simulink model "testAlphaWallOut"  (R2013b)
settings: Solver=VariableStepDiscrete  StartTime=0.0  StopTime=20  RelTol=1e-3
libraries: carnot x3, simulink x1
settings Model: Creator=drhf  LastModifiedBy=drhf
settings DataIOCC: ReturnWorkspaceOutputs=on
settings OptimizationCC: InlineParams=on
settings DebuggingCC: ReadBeforeWriteMsg=DisableAll  WriteAfterWriteMsg=DisableAll  WriteAfterReadMsg=DisableAll  MultiTaskDSMMsg=none
settings ModelReferenceCC: UpdateModelReferenceTargets=IfOutOfDate
settings SFSimCC: SFSimEcho=off

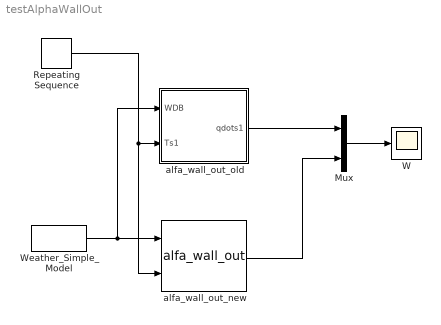
== system testAlphaWallOut ==
  Mux : Mux  Inputs=2
  Repeating Sequence : simulink/Sources/Repeating Sequence  rep_seq_t=[0 10]  rep_seq_y=[10 30]
  W : Scope
  Weather_Simple_Model : carnot/Weather/Weather_Simple_Model  lat=60  Ibn=900  Idg=100  tamb=5  deltaTsky=-6  rh=50  precip="10e-3/24/3600           % 10 mm in 24 h"  cloud=0.125  p=1013e2  vw=1  wdir=270
  alfa_wall_out_new : carnot/Load/Houses/heat_transfer/alfa_wall_out  pos=0  absorption_out=0.4  emission_out=0.7  wallsurface=1
  alfa_wall_out_old : Subsystem  AncestorBlock=carnot/Load/Houses/heat_transfer/alfa_wall_out  mask(ALFA){pos=0, absorption_out=0.4, emission_out=0.7, wallsurface=1}
      mask prompts: pos "Azimut (south = 0, east = -90) in degrees"; absorption_out "Solar absorption outside (0..1)"; emission_out "Longwave emissivity of surface (0..1)"; wallsurface "Wall surface in m²"
      mask help:
      | Convective and radiative HEAT TRANSFER at the WEATHER EXPOSED SURFACE of an OUTER WALL.
      |
      | [W*] : modified weather data, adapted to height over ground,
      | Ts : temperature of outdoor wall surface, °C,
      | qdots : specific heat flow into wall / window construction, W/m^2.
      mask init:
      | if length(pos) == 1
      |     pos = [90  pos 0]; % pos is [inclination azimut rotation]
      | end
  wires:
  Repeating Sequence/1 -> alfa_wall_out_old/2(Ts1), alfa_wall_out_new/2
  alfa_wall_out_old/1(qdots1) -> Mux/1
  alfa_wall_out_new/1 -> Mux/2
  Mux/1 -> W/1
  Weather_Simple_Model/1 -> alfa_wall_out_old/1(WDB), alfa_wall_out_new/1

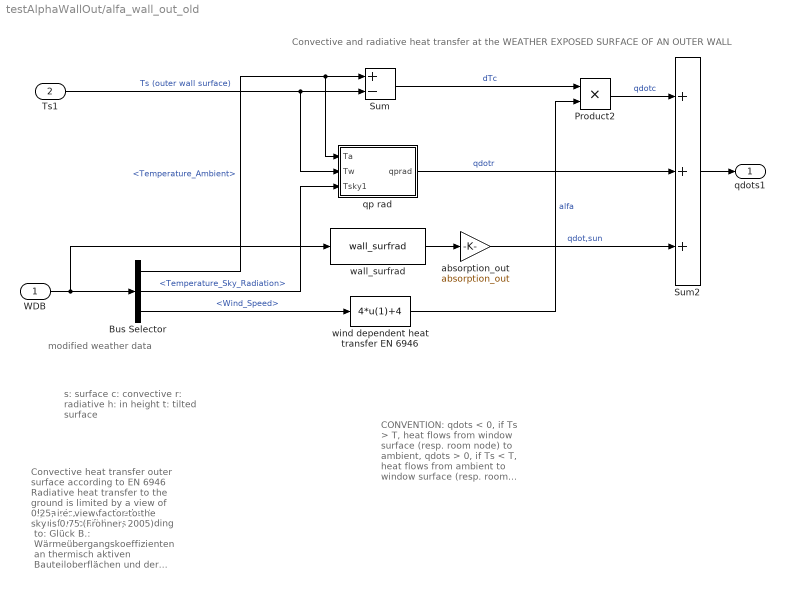
== system testAlphaWallOut/alfa_wall_out_old ==
  note: dynamic, convective heat transfer coefficients according to: Glück B.: Wärmeübergangskoeffizienten an thermisch aktiven Bauteiloberflächen
      | und der Übergang zu Basiskennlinien für die Wärmestromdichte; gi Gesundheits-Ingenieur; 128. Jahrgang 2007, Heft 1, Seiten 1-10
  note: Convective heat transfer outer surface according to EN 6946
      | Radiative heat transfer to the ground is limited by a view of 0.25, i.e. view factor to the sky is 0.75 (Frohner, 2005)
  note: Convective and radiative heat transfer at the WEATHER EXPOSED SURFACE OF AN OUTER WALL
  note: s: surface
      | c: convective
      | r: radiative
      | h: in height
      | t: tilted surface
  note: modified
      | weather data
  note: CONVENTION:
      | qdots < 0, if Ts > T, heat flows from window surface (resp. room node) to ambient,
      | qdots > 0, if Ts < T, heat flows from ambient to window surface (resp. room node).
  WDB : Inport
  Ts1 : Inport  Port=2
  Bus Selector : BusSelector  OutputSignals=Temperature_Ambient,Temperature_Sky_Radiation,Wind_Speed
  Product2 : Product  SaturateOnIntegerOverflow=on  RndMeth=Zero  InputSameDT=on  OutDataTypeStr=Inherit: Same as first input
  Sum : Sum  Inputs=+-  SaturateOnIntegerOverflow=on  InputSameDT=on  OutDataTypeStr=Inherit: Same as first input
  Sum2 : Sum  Inputs=+++  SaturateOnIntegerOverflow=on  InputSameDT=on  OutDataTypeStr=Inherit: Same as first input
  absorption_out : Gain  Gain=absorption_out  SaturateOnIntegerOverflow=on  OutDataTypeStr=Inherit: Same as input  ParamDataTypeStr=Inherit: Same as input
  qp rad : Subsystem
  wall_surfrad : carnot/Load/Houses/heat_transfer/wall_surfrad  pos=pos
  wind dependent heat transfer EN 6946 : Fcn  Expr=4*u(1)+4
  qdots1 : Outport
  wires:
  Bus Selector/3 -> wind dependent heat transfer EN 6946/1  "<Wind_Speed>"
  Bus Selector/2 -> qp rad/3(Tsky1)  "<Temperature_Sky_Radiation>"
  Bus Selector/1 -> qp rad/1(Ta), Sum/1  "<Temperature_Ambient>"
  Sum/1 -> Product2/1  "dTc"
  WDB/1 -> wall_surfrad/1, Bus Selector/1
  Sum2/1 -> qdots1/1
  Ts1/1 -> Sum/2, qp rad/2(Tw)  "Ts (outer wall surface)"
  wall_surfrad/1 -> absorption_out/1
  wind dependent heat transfer EN 6946/1 -> Product2/2  "alfa"
  absorption_out/1 -> Sum2/3  "qdot,sun"
  Product2/1 -> Sum2/1  "qdotc"
  qp rad/1(qprad) -> Sum2/2  "qdotr"

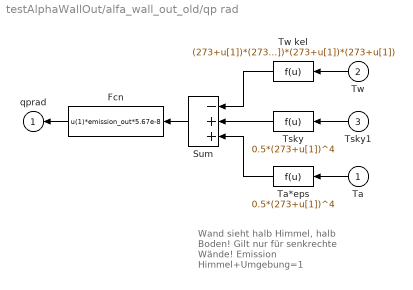
== system testAlphaWallOut/alfa_wall_out_old/qp rad ==
  note: Wand sieht halb Himmel, halb Boden! Gilt nur für senkrechte Wände!
      | Emission Himmel+Umgebung=1
  Ta : Inport
  Tw : Inport  Port=2
  Tsky1 : Inport  Port=3
  Fcn : Fcn  Expr=u(1)*emission_out*5.67e-8
  Sum : Sum  Inputs=-++  SaturateOnIntegerOverflow=on  InputSameDT=on  OutDataTypeStr=Inherit: Same as first input
  Ta*eps : Fcn  Expr=0.5*(273+u[1])^4
  Tsky : Fcn  Expr=0.5*(273+u[1])^4
  Tw kel : Fcn  Expr=(273+u[1])*(273+u[1])*(273+u[1])*(273+u[1])
  qprad : Outport
  wires:
  Tsky/1 -> Sum/2
  Tw kel/1 -> Sum/1
  Tw/1 -> Tw kel/1
  Ta*eps/1 -> Sum/3
  Sum/1 -> Fcn/1
  Fcn/1 -> qprad/1
  Ta/1 -> Ta*eps/1
  Tsky1/1 -> Tsky/1
